simulink model "gg_plus_lc_platoon"  (R2019a)
settings: Solver=ode23t  StartTime=0.0  StopTime=70  FixedStep=0.1  MaxStep=0.01  RelTol=1e-3
InitFcn:
  | load vehStatesBus
libraries: simulink x120, powerlib_meascontrol x14, dspsigops x7, autolibshared x7
(part 7 of 7)

== system gg_plus_lc_platoon/p3/Virtual Vehicle Following/Virtual Leader Following ==
  eh : Inport
  ev : Inport  Port=2
  realInput : Inport  Port=3
  intReset : Inport  Port=4
  Anti-windup gain : Gain  Gain=sqrt(Ki/Kd)
  Gain : Gain  Gain=10
  Integrator : Integrator  ExternalReset=rising
  Integrator2 : Integrator  ExternalReset=rising
  Kd : Gain  Gain=Kd
  Ki : Gain  Gain=Ki
  Kp : Gain  Gain=Kp
  Saturation1 : Saturate  UpperLimit=maxHeadwayError  LowerLimit=minHeadwayError
  Scope : Scope  NumInputPorts=4
  Scope1 : Scope  NumInputPorts=2
  Sum : Sum  Inputs=|-+
  Sum1 : Sum  Inputs=+++
  Sum5 : Sum  Inputs=-+|
  Sum9 : Sum  Inputs=|+-
  u : Outport
  wires:
  Saturation1/1 -> Sum9/1, Scope1/1
  Sum9/1 -> Gain/1
  Gain/1 -> Integrator2/1
  ev/1 -> Kd/1
  Ki/1 -> Sum5/2
  Anti-windup gain/1 -> Sum5/1
  Sum5/1 -> Integrator/1
  Integrator/1 -> Sum1/1, Scope/1
  Kp/1 -> Scope/2, Sum1/2
  Kd/1 -> Scope/3, Sum1/3
  Integrator2/1 -> Kp/1, Ki/1, Scope1/2, Sum9/2
  eh/1 -> Saturation1/1
  Sum1/1 -> Sum/2, u/1, Scope/4
  realInput/1 -> Sum/1
  Sum/1 -> Anti-windup gain/1
  intReset/1 -> Integrator/2, Integrator2/2

== system gg_plus_lc_platoon/p3/findLeader/Subsystem ==
  ego : Inport
  all : Inport  Port=2
  Enable : EnablePort
  MATLAB Function : MATLAB Function  TreatAsAtomicUnit=on
  idx : Outport  InitialOutput=1
  wires:
  ego/1 -> MATLAB Function/1(ego)
  MATLAB Function/1(leaderIdx) -> idx/1
  all/1 -> MATLAB Function/2(allVehicles)

== system gg_plus_lc_platoon/p3/findLeader/farAwayVeh ==
  ego : Inport  OutDataTypeStr=Bus: vehStatesBus
  Bus Creator : BusCreator  Inputs=6  OutDataTypeStr=Bus: vehStatesBus  NonVirtualBus=on
  Bus Selector : BusSelector  OutputSignals=X,Y,Xdot,psi,u,delta
  Constant : Constant  Value=1000
  Sum : Sum  Inputs=++|
  Out1 : Outport  OutDataTypeStr=Bus: vehStatesBus
  wires:
  Bus Creator/1 -> Out1/1
  Constant/1 -> Sum/1
  Bus Selector/1 -> Sum/2  "<X>"
  ego/1 -> Bus Selector/1
  Sum/1 -> Bus Creator/1  "X"
  Bus Selector/2 -> Bus Creator/2  "<Y>"
  Bus Selector/3 -> Bus Creator/3  "<Xdot>"
  Bus Selector/4 -> Bus Creator/4  "<psi>"
  Bus Selector/5 -> Bus Creator/5  "<u>"
  Bus Selector/6 -> Bus Creator/6  "<delta>"

== system gg_plus_lc_platoon/p3/followerErrors/gapToFollower ==
  xf : Inport
  vf : Inport  Port=2
  xl : Inport  Port=3
  Multiply : Product
  Sum : Sum  Inputs=-+|
  Sum1 : Sum  Inputs=++|
  Sum2 : Sum  Inputs=+-|
  Sum3 : Sum  Inputs=|++
  d0 : Constant  Value=d0
  h : Constant  Value=h
  vLen : Constant  Value=lr+lf
  eh : Outport
  "gap " : Outport  Port=2
  wires:
  vLen/1 -> Sum1/1
  Multiply/1 -> Sum3/1
  Sum/1 -> "gap "/1, Sum2/1  "gap"
  xf/1 -> Sum1/2
  Sum3/1 -> Sum2/2  "desired  gap"
  vf/1 -> Multiply/1
  Sum1/1 -> Sum/1  "x (front bumber)"
  xl/1 -> Sum/2
  Sum2/1 -> eh/1
  h/1 -> Multiply/2  "time headway"
  d0/1 -> Sum3/2  "gap at  standstill"

== system gg_plus_lc_platoon/p3/safeErrors/Triggered Subsystem1 ==
  Trigger : TriggerPort  VariantControl=Variant
  Constant : Constant  Value=true  OutDataTypeStr=boolean
  Out1 : Outport  OutDataTypeStr=boolean  InitialOutput=0
  wires:
  Constant/1 -> Out1/1

== matlab function gg_plus_lc_platoon/Lo/Subsystem2/MATLAB Function ==
  data: strategy input; longAdjFlag output; posInPlatoon input; platoonState input
function longAdjFlag = startLongAdjustment(strategy, posInPlatoon, platoonState)

switch strategy
    case {1, 2}
        if posInPlatoon == 1
            longAdjFlag = true;
        else
            longAdjFlag = platoonState(posInPlatoon-1)>1;
        end
    case 3
        if posInPlatoon == length(platoonState)
            longAdjFlag = true;
        else
           longAdjFlag = platoonState(posInPlatoon+1)>4;
        end 
    otherwise
        error('Unknown strategy')
end

== matlab function gg_plus_lc_platoon/p1/Subsystem2/MATLAB Function ==
  data: strategy input; longAdjFlag output; posInPlatoon input; platoonState input
function longAdjFlag = startLongAdjustment(strategy, posInPlatoon, platoonState)

switch strategy
    case {1, 2}
        if posInPlatoon == 1
            longAdjFlag = true;
        else
            longAdjFlag = platoonState(posInPlatoon-1)>1;
        end
    case 3
        if posInPlatoon == length(platoonState)
            longAdjFlag = true;
        else
           longAdjFlag = platoonState(posInPlatoon+1)>4;
        end 
    otherwise
        error('Unknown strategy')
end

== stateflow chart gg_plus_lc_platoon/Lo/Virtual Vehicle Following/Chart ==
  state SpeedControlFreeFlow
    entry:
    state=2;
    during:
    u = uFreeFlowVelControl;
  state VehFollowing
    entry:
    state=0;
    during:
    u = uVehFoll;
  state SpeedControlMin
    entry:
    state = 1;
    during:
    u = uMinVelControl;
  (default) -> VehFollowing
  VehFollowing -> SpeedControlFreeFlow [order 2] : [~leaderWithinRange]
  SpeedControlFreeFlow -> VehFollowing : [leaderWithinRange]
  VehFollowing -> SpeedControlMin [order 1] : [(velDiff>=0) && (uVehFoll<0)]
  SpeedControlMin -> VehFollowing : [uVehFoll>=uMinVelControl]
  data: uFreeFlowVelControl input; leaderWithinRange input; uVehFoll input size=1; state output size=1; u output size=1; velDiff input size=1; uMinVelControl input double

== stateflow chart gg_plus_lc_platoon/Lo/controlChoice/ControlChoice ==
  state RegVehFoll
    during:
    data = regVehFollData;
  state AdjForLaneChange
    during:
    if ~xor(leaderInRange, vLeaderInRange)
    data = min(regVehFollData, longAdjustmentData);
    elseif vLeaderInRange
    data = longAdjustmentData;
    else
    data = regVehFollData;
    end
  (default) -> RegVehFoll
  RegVehFoll -> AdjForLaneChange : [state==1]
  data: state input; leaderInRange input; regVehFollData input; data output; longAdjustmentData input; vLeaderInRange input

== matlab function gg_plus_lc_platoon/Lo/findLeader/Subsystem/MATLAB Function ==
  data: ego input Bus: vehStatesBus; allVehicles input; leaderIdx output
function leaderIdx  = findLeader(ego, allVehicles)

nv = length(allVehicles);

leaderIdx = nv+1;

farAwayVehicle.X = ego.X + 10^4;
farAwayVehicle.Y = ego.Y;
farAwayVehicle.Xdot = ego.Xdot;
farAwayVehicle.u = 0;

leader = farAwayVehicle;
% For non lane changing vehicles, the leader is whoever is longitudinally
% closer and with any part of the body in the same lane.
% 1.8m (half lane) + 0.9m (half veh width)
for n = 1:nv
    if allVehicles(n).X>ego.X
        if abs(allVehicles(n).Y - ego.Y)<=2.7 && allVehicles(n).X<leader.X
            leaderIdx = n;
        end
    end
end

== matlab function gg_plus_lc_platoon/Lo/virtualVehiclesManager/MATLAB Function ==
  data: nVehicles input; longAdj input; lcFlag input; lcDone input; virtualLeaderIdx output; posInPlatoon input; lcStrategy input
function virtualLeaderIdx  = ...
    determineVirtualLeader(nVehicles, longAdj, lcFlag, lcDone, posInPlatoon, lcStrategy)

% Important assumption:
% The array of vehicles is ordered as [Ld, Fd, Lo, p1, ..., pN, Fo]

% To consider: would it be more organized to have two vehicle arrays (one 
% for each lane)?

if ~longAdj % vehicle not involved in LC
    virtualLeaderIdx = 1;
    return
end

if ~lcFlag% gap generating vehicle
    virtualLeaderIdx = nVehicles-1; % last platoon vehicle
    
else % lane changing vehicle
    switch lcStrategy
        case {1, 2} % synchronous, leader changes first
            if posInPlatoon == 1
                virtualLeaderIdx = 1;
            else
                virtualLeaderIdx = 3 + (posInPlatoon - 1);
            end
            
        case 3 % last veh changes first
            if ~lcDone
                virtualLeaderIdx = 1;
            else
                if posInPlatoon == 1
                    virtualLeaderIdx = 1;
                else
                    virtualLeaderIdx = 3 + (posInPlatoon - 1);
                end
            end
            
        otherwise
            error('[determineVirtualLeader in Simulink model] Unknown lane changing strategy]')
    end
end

end

== matlab function gg_plus_lc_platoon/Lo/virtualVehiclesManager/MATLAB Function1 ==
  data: nVehicles input; longAdj input; lcFlag input; posInPlatoon input; lcStrategy input; virtualFollowerIdx output
function virtualFollowerIdx  = ...
    determineVirtualFollower(nVehicles, longAdj, lcFlag, posInPlatoon, lcStrategy)

% Important assumption:
% The array of vehicles is ordered as [Ld, Fd, Lo, p1, ..., pN, Fo]

% To consider: would it be more organized to have two vehicle arrays (one 
% for each lane)?

if ~longAdj % vehicle not involved in LC
    virtualFollowerIdx = nVehicles;
    return
end

if ~lcFlag% gap generating vehicle
    virtualFollowerIdx = nVehicles;
    
else % lane changing vehicle
    switch lcStrategy
        case {1, 2} % synchronous, leader changes first
            virtualFollowerIdx = 2;
        case 3 % last veh changes first
            if posInPlatoon == nVehicles-4
                virtualFollowerIdx = 2;
            else
                virtualFollowerIdx = 3 + (posInPlatoon + 1);
            end
        otherwise
            error('[determineVirtualFollower in Simulink model] Unknown lane changing strategy]')
    end
end

end

== matlab function gg_plus_lc_platoon/Fo/Subsystem2/MATLAB Function ==
  data: strategy input; longAdjFlag output; posInPlatoon input; platoonState input
function longAdjFlag = startLongAdjustment(strategy, posInPlatoon, platoonState)

switch strategy
    case {1, 2}
        if posInPlatoon == 1
            longAdjFlag = true;
        else
            longAdjFlag = platoonState(posInPlatoon-1)>1;
        end
    case 3
        if posInPlatoon == length(platoonState)
            longAdjFlag = true;
        else
           longAdjFlag = platoonState(posInPlatoon+1)>4;
        end 
    otherwise
        error('Unknown strategy')
end

== stateflow chart gg_plus_lc_platoon/Fo/Virtual Vehicle Following/Chart ==
  state SpeedControlFreeFlow
    entry:
    state=2;
    during:
    u = uFreeFlowVelControl;
  state VehFollowing
    entry:
    state=0;
    during:
    u = uVehFoll;
  state SpeedControlMin
    entry:
    state = 1;
    during:
    u = uMinVelControl;
  (default) -> VehFollowing
  VehFollowing -> SpeedControlFreeFlow [order 2] : [~leaderWithinRange]
  SpeedControlFreeFlow -> VehFollowing : [leaderWithinRange]
  VehFollowing -> SpeedControlMin [order 1] : [(velDiff>=0) && (uVehFoll<0)]
  SpeedControlMin -> VehFollowing : [uVehFoll>=uMinVelControl]
  data: uFreeFlowVelControl input; leaderWithinRange input; uVehFoll input size=1; state output size=1; u output size=1; velDiff input size=1; uMinVelControl input double

== stateflow chart gg_plus_lc_platoon/Fo/controlChoice/ControlChoice ==
  state RegVehFoll
    during:
    data = regVehFollData;
  state AdjForLaneChange
    during:
    if ~xor(leaderInRange, vLeaderInRange)
    data = min(regVehFollData, longAdjustmentData);
    elseif vLeaderInRange
    data = longAdjustmentData;
    else
    data = regVehFollData;
    end
  (default) -> RegVehFoll
  RegVehFoll -> AdjForLaneChange : [state==1]
  data: state input; leaderInRange input; regVehFollData input; data output; longAdjustmentData input; vLeaderInRange input

== matlab function gg_plus_lc_platoon/Fo/findLeader/Subsystem/MATLAB Function ==
  data: ego input Bus: vehStatesBus; allVehicles input; leaderIdx output
function leaderIdx  = findLeader(ego, allVehicles)

nv = length(allVehicles);

leaderIdx = nv+1;

farAwayVehicle.X = ego.X + 10^4;
farAwayVehicle.Y = ego.Y;
farAwayVehicle.Xdot = ego.Xdot;
farAwayVehicle.u = 0;

leader = farAwayVehicle;
% For non lane changing vehicles, the leader is whoever is longitudinally
% closer and with any part of the body in the same lane.
% 1.8m (half lane) + 0.9m (half veh width)
for n = 1:nv
    if allVehicles(n).X>ego.X
        if abs(allVehicles(n).Y - ego.Y)<=2.7 && allVehicles(n).X<leader.X
            leaderIdx = n;
        end
    end
end

== matlab function gg_plus_lc_platoon/Fo/virtualVehiclesManager/MATLAB Function ==
  data: nVehicles input; longAdj input; lcFlag input; lcDone input; virtualLeaderIdx output; posInPlatoon input; lcStrategy input
function virtualLeaderIdx  = ...
    determineVirtualLeader(nVehicles, longAdj, lcFlag, lcDone, posInPlatoon, lcStrategy)

% Important assumption:
% The array of vehicles is ordered as [Ld, Fd, Lo, p1, ..., pN, Fo]

% To consider: would it be more organized to have two vehicle arrays (one 
% for each lane)?

if ~longAdj % vehicle not involved in LC
    virtualLeaderIdx = 1;
    return
end

if ~lcFlag% gap generating vehicle
    virtualLeaderIdx = nVehicles-1; % last platoon vehicle
    
else % lane changing vehicle
    switch lcStrategy
        case {1, 2} % synchronous, leader changes first
            if posInPlatoon == 1
                virtualLeaderIdx = 1;
            else
                virtualLeaderIdx = 3 + (posInPlatoon - 1);
            end
            
        case 3 % last veh changes first
            if ~lcDone
                virtualLeaderIdx = 1;
            else
                if posInPlatoon == 1
                    virtualLeaderIdx = 1;
                else
                    virtualLeaderIdx = 3 + (posInPlatoon - 1);
                end
            end
            
        otherwise
            error('[determineVirtualLeader in Simulink model] Unknown lane changing strategy]')
    end
end

end

== matlab function gg_plus_lc_platoon/Fo/virtualVehiclesManager/MATLAB Function1 ==
  data: nVehicles input; longAdj input; lcFlag input; posInPlatoon input; lcStrategy input; virtualFollowerIdx output
function virtualFollowerIdx  = ...
    determineVirtualFollower(nVehicles, longAdj, lcFlag, posInPlatoon, lcStrategy)

% Important assumption:
% The array of vehicles is ordered as [Ld, Fd, Lo, p1, ..., pN, Fo]

% To consider: would it be more organized to have two vehicle arrays (one 
% for each lane)?

if ~longAdj % vehicle not involved in LC
    virtualFollowerIdx = nVehicles;
    return
end

if ~lcFlag% gap generating vehicle
    virtualFollowerIdx = nVehicles;
    
else % lane changing vehicle
    switch lcStrategy
        case {1, 2} % synchronous, leader changes first
            virtualFollowerIdx = 2;
        case 3 % last veh changes first
            if posInPlatoon == nVehicles-4
                virtualFollowerIdx = 2;
            else
                virtualFollowerIdx = 3 + (posInPlatoon + 1);
            end
        otherwise
            error('[determineVirtualFollower in Simulink model] Unknown lane changing strategy]')
    end
end

end

== stateflow chart gg_plus_lc_platoon/p1/Virtual Vehicle Following/Chart ==
  state SpeedControlFreeFlow
    entry:
    state=2;
    during:
    u = uFreeFlowVelControl;
  state VehFollowing
    entry:
    state=0;
    during:
    u = uVehFoll;
  state SpeedControlMin
    entry:
    state = 1;
    during:
    u = uMinVelControl;
  (default) -> VehFollowing
  VehFollowing -> SpeedControlFreeFlow [order 2] : [~leaderWithinRange]
  SpeedControlFreeFlow -> VehFollowing : [leaderWithinRange]
  VehFollowing -> SpeedControlMin [order 1] : [(velDiff>=0) && (uVehFoll<0)]
  SpeedControlMin -> VehFollowing : [uVehFoll>=uMinVelControl]
  data: uFreeFlowVelControl input; leaderWithinRange input; uVehFoll input size=1; state output size=1; u output size=1; velDiff input size=1; uMinVelControl input double

== stateflow chart gg_plus_lc_platoon/p1/controlChoice/ControlChoice ==
  state RegVehFoll
    during:
    data = regVehFollData;
  state AdjForLaneChange
    during:
    if ~xor(leaderInRange, vLeaderInRange)
    data = min(regVehFollData, longAdjustmentData);
    elseif vLeaderInRange
    data = longAdjustmentData;
    else
    data = regVehFollData;
    end
  (default) -> RegVehFoll
  RegVehFoll -> AdjForLaneChange : [state==1]
  data: state input; leaderInRange input; regVehFollData input; data output; longAdjustmentData input; vLeaderInRange input

== matlab function gg_plus_lc_platoon/p1/findLeader/Subsystem/MATLAB Function ==
  data: ego input Bus: vehStatesBus; allVehicles input; leaderIdx output
function leaderIdx  = findLeader(ego, allVehicles)

nv = length(allVehicles);

leaderIdx = nv+1;

farAwayVehicle.X = ego.X + 10^4;
farAwayVehicle.Y = ego.Y;
farAwayVehicle.Xdot = ego.Xdot;
farAwayVehicle.u = 0;

leader = farAwayVehicle;
% For non lane changing vehicles, the leader is whoever is longitudinally
% closer and with any part of the body in the same lane.
% 1.8m (half lane) + 0.9m (half veh width)
for n = 1:nv
    if allVehicles(n).X>ego.X
        if abs(allVehicles(n).Y - ego.Y)<=2.7 && allVehicles(n).X<leader.X
            leaderIdx = n;
        end
    end
end

== matlab function gg_plus_lc_platoon/p1/virtualVehiclesManager/MATLAB Function ==
  data: nVehicles input; longAdj input; lcFlag input; lcDone input; virtualLeaderIdx output; posInPlatoon input; lcStrategy input
function virtualLeaderIdx  = ...
    determineVirtualLeader(nVehicles, longAdj, lcFlag, lcDone, posInPlatoon, lcStrategy)

% Important assumption:
% The array of vehicles is ordered as [Ld, Fd, Lo, p1, ..., pN, Fo]

% To consider: would it be more organized to have two vehicle arrays (one 
% for each lane)?

if ~longAdj % vehicle not involved in LC
    virtualLeaderIdx = 1;
    return
end

if ~lcFlag% gap generating vehicle
    virtualLeaderIdx = nVehicles-1; % last platoon vehicle
    
else % lane changing vehicle
    switch lcStrategy
        case {1, 2} % synchronous, leader changes first
            if posInPlatoon == 1
                virtualLeaderIdx = 1;
            else
                virtualLeaderIdx = 3 + (posInPlatoon - 1);
            end
            
        case 3 % last veh changes first
            if ~lcDone
                virtualLeaderIdx = 1;
            else
                if posInPlatoon == 1
                    virtualLeaderIdx = 1;
                else
                    virtualLeaderIdx = 3 + (posInPlatoon - 1);
                end
            end
            
        otherwise
            error('[determineVirtualLeader in Simulink model] Unknown lane changing strategy]')
    end
end

end

== matlab function gg_plus_lc_platoon/p1/virtualVehiclesManager/MATLAB Function1 ==
  data: nVehicles input; longAdj input; lcFlag input; posInPlatoon input; lcStrategy input; virtualFollowerIdx output
function virtualFollowerIdx  = ...
    determineVirtualFollower(nVehicles, longAdj, lcFlag, posInPlatoon, lcStrategy)

% Important assumption:
% The array of vehicles is ordered as [Ld, Fd, Lo, p1, ..., pN, Fo]

% To consider: would it be more organized to have two vehicle arrays (one 
% for each lane)?

if ~longAdj % vehicle not involved in LC
    virtualFollowerIdx = nVehicles;
    return
end

if ~lcFlag% gap generating vehicle
    virtualFollowerIdx = nVehicles;
    
else % lane changing vehicle
    switch lcStrategy
        case {1, 2} % synchronous, leader changes first
            virtualFollowerIdx = 2;
        case 3 % last veh changes first
            if posInPlatoon == nVehicles-4
                virtualFollowerIdx = 2;
            else
                virtualFollowerIdx = 3 + (posInPlatoon + 1);
            end
        otherwise
            error('[determineVirtualFollower in Simulink model] Unknown lane changing strategy]')
    end
end

end

== matlab function gg_plus_lc_platoon/p2/Subsystem2/MATLAB Function ==
  data: strategy input; longAdjFlag output; posInPlatoon input; platoonState input
function longAdjFlag = startLongAdjustment(strategy, posInPlatoon, platoonState)

switch strategy
    case {1, 2}
        if posInPlatoon == 1
            longAdjFlag = true;
        else
            longAdjFlag = platoonState(posInPlatoon-1)>1;
        end
    case 3
        if posInPlatoon == length(platoonState)
            longAdjFlag = true;
        else
           longAdjFlag = platoonState(posInPlatoon+1)>4;
        end 
    otherwise
        error('Unknown strategy')
end

== stateflow chart gg_plus_lc_platoon/p2/Virtual Vehicle Following/Chart ==
  state SpeedControlFreeFlow
    entry:
    state=2;
    during:
    u = uFreeFlowVelControl;
  state VehFollowing
    entry:
    state=0;
    during:
    u = uVehFoll;
  state SpeedControlMin
    entry:
    state = 1;
    during:
    u = uMinVelControl;
  (default) -> VehFollowing
  VehFollowing -> SpeedControlFreeFlow [order 2] : [~leaderWithinRange]
  SpeedControlFreeFlow -> VehFollowing : [leaderWithinRange]
  VehFollowing -> SpeedControlMin [order 1] : [(velDiff>=0) && (uVehFoll<0)]
  SpeedControlMin -> VehFollowing : [uVehFoll>=uMinVelControl]
  data: uFreeFlowVelControl input; leaderWithinRange input; uVehFoll input size=1; state output size=1; u output size=1; velDiff input size=1; uMinVelControl input double

== stateflow chart gg_plus_lc_platoon/p2/controlChoice/ControlChoice ==
  state RegVehFoll
    during:
    data = regVehFollData;
  state AdjForLaneChange
    during:
    if ~xor(leaderInRange, vLeaderInRange)
    data = min(regVehFollData, longAdjustmentData);
    elseif vLeaderInRange
    data = longAdjustmentData;
    else
    data = regVehFollData;
    end
  (default) -> RegVehFoll
  RegVehFoll -> AdjForLaneChange : [state==1]
  data: state input; leaderInRange input; regVehFollData input; data output; longAdjustmentData input; vLeaderInRange input

== matlab function gg_plus_lc_platoon/p2/findLeader/Subsystem/MATLAB Function ==
  data: ego input Bus: vehStatesBus; allVehicles input; leaderIdx output
function leaderIdx  = findLeader(ego, allVehicles)

nv = length(allVehicles);

leaderIdx = nv+1;

farAwayVehicle.X = ego.X + 10^4;
farAwayVehicle.Y = ego.Y;
farAwayVehicle.Xdot = ego.Xdot;
farAwayVehicle.u = 0;

leader = farAwayVehicle;
% For non lane changing vehicles, the leader is whoever is longitudinally
% closer and with any part of the body in the same lane.
% 1.8m (half lane) + 0.9m (half veh width)
for n = 1:nv
    if allVehicles(n).X>ego.X
        if abs(allVehicles(n).Y - ego.Y)<=2.7 && allVehicles(n).X<leader.X
            leaderIdx = n;
        end
    end
end

== matlab function gg_plus_lc_platoon/p2/virtualVehiclesManager/MATLAB Function ==
  data: nVehicles input; longAdj input; lcFlag input; lcDone input; virtualLeaderIdx output; posInPlatoon input; lcStrategy input
function virtualLeaderIdx  = ...
    determineVirtualLeader(nVehicles, longAdj, lcFlag, lcDone, posInPlatoon, lcStrategy)

% Important assumption:
% The array of vehicles is ordered as [Ld, Fd, Lo, p1, ..., pN, Fo]

% To consider: would it be more organized to have two vehicle arrays (one 
% for each lane)?

if ~longAdj % vehicle not involved in LC
    virtualLeaderIdx = 1;
    return
end

if ~lcFlag% gap generating vehicle
    virtualLeaderIdx = nVehicles-1; % last platoon vehicle
    
else % lane changing vehicle
    switch lcStrategy
        case {1, 2} % synchronous, leader changes first
            if posInPlatoon == 1
                virtualLeaderIdx = 1;
            else
                virtualLeaderIdx = 3 + (posInPlatoon - 1);
            end
            
        case 3 % last veh changes first
            if ~lcDone
                virtualLeaderIdx = 1;
            else
                if posInPlatoon == 1
                    virtualLeaderIdx = 1;
                else
                    virtualLeaderIdx = 3 + (posInPlatoon - 1);
                end
            end
            
        otherwise
            error('[determineVirtualLeader in Simulink model] Unknown lane changing strategy]')
    end
end

end

== matlab function gg_plus_lc_platoon/Fd/Subsystem2/MATLAB Function ==
  data: strategy input; longAdjFlag output; posInPlatoon input; platoonState input
function longAdjFlag = startLongAdjustment(strategy, posInPlatoon, platoonState)

switch strategy
    case {1, 2}
        if posInPlatoon == 1
            longAdjFlag = true;
        else
            longAdjFlag = platoonState(posInPlatoon-1)>1;
        end
    case 3
        if posInPlatoon == length(platoonState)
            longAdjFlag = true;
        else
           longAdjFlag = platoonState(posInPlatoon+1)>4;
        end 
    otherwise
        error('Unknown strategy')
end

== matlab function gg_plus_lc_platoon/p2/virtualVehiclesManager/MATLAB Function1 ==
  data: nVehicles input; longAdj input; lcFlag input; posInPlatoon input; lcStrategy input; virtualFollowerIdx output
function virtualFollowerIdx  = ...
    determineVirtualFollower(nVehicles, longAdj, lcFlag, posInPlatoon, lcStrategy)

% Important assumption:
% The array of vehicles is ordered as [Ld, Fd, Lo, p1, ..., pN, Fo]

% To consider: would it be more organized to have two vehicle arrays (one 
% for each lane)?

if ~longAdj % vehicle not involved in LC
    virtualFollowerIdx = nVehicles;
    return
end

if ~lcFlag% gap generating vehicle
    virtualFollowerIdx = nVehicles;
    
else % lane changing vehicle
    switch lcStrategy
        case {1, 2} % synchronous, leader changes first
            virtualFollowerIdx = 2;
        case 3 % last veh changes first
            if posInPlatoon == nVehicles-4
                virtualFollowerIdx = 2;
            else
                virtualFollowerIdx = 3 + (posInPlatoon + 1);
            end
        otherwise
            error('[determineVirtualFollower in Simulink model] Unknown lane changing strategy]')
    end
end

end

== matlab function gg_plus_lc_platoon/p3/Subsystem2/MATLAB Function ==
  data: strategy input; longAdjFlag output; posInPlatoon input; platoonState input
function longAdjFlag = startLongAdjustment(strategy, posInPlatoon, platoonState)

switch strategy
    case {1, 2}
        if posInPlatoon == 1
            longAdjFlag = true;
        else
            longAdjFlag = platoonState(posInPlatoon-1)>1;
        end
    case 3
        if posInPlatoon == length(platoonState)
            longAdjFlag = true;
        else
           longAdjFlag = platoonState(posInPlatoon+1)>4;
        end 
    otherwise
        error('Unknown strategy')
end

== stateflow chart gg_plus_lc_platoon/p3/Virtual Vehicle Following/Chart ==
  state SpeedControlFreeFlow
    entry:
    state=2;
    during:
    u = uFreeFlowVelControl;
  state VehFollowing
    entry:
    state=0;
    during:
    u = uVehFoll;
  state SpeedControlMin
    entry:
    state = 1;
    during:
    u = uMinVelControl;
  (default) -> VehFollowing
  VehFollowing -> SpeedControlFreeFlow [order 2] : [~leaderWithinRange]
  SpeedControlFreeFlow -> VehFollowing : [leaderWithinRange]
  VehFollowing -> SpeedControlMin [order 1] : [(velDiff>=0) && (uVehFoll<0)]
  SpeedControlMin -> VehFollowing : [uVehFoll>=uMinVelControl]
  data: uFreeFlowVelControl input; leaderWithinRange input; uVehFoll input size=1; state output size=1; u output size=1; velDiff input size=1; uMinVelControl input double

== stateflow chart gg_plus_lc_platoon/p3/controlChoice/ControlChoice ==
  state RegVehFoll
    during:
    data = regVehFollData;
  state AdjForLaneChange
    during:
    if ~xor(leaderInRange, vLeaderInRange)
    data = min(regVehFollData, longAdjustmentData);
    elseif vLeaderInRange
    data = longAdjustmentData;
    else
    data = regVehFollData;
    end
  (default) -> RegVehFoll
  RegVehFoll -> AdjForLaneChange : [state==1]
  data: state input; leaderInRange input; regVehFollData input; data output; longAdjustmentData input; vLeaderInRange input

== matlab function gg_plus_lc_platoon/p3/findLeader/Subsystem/MATLAB Function ==
  data: ego input Bus: vehStatesBus; allVehicles input; leaderIdx output
function leaderIdx  = findLeader(ego, allVehicles)

nv = length(allVehicles);

leaderIdx = nv+1;

farAwayVehicle.X = ego.X + 10^4;
farAwayVehicle.Y = ego.Y;
farAwayVehicle.Xdot = ego.Xdot;
farAwayVehicle.u = 0;

leader = farAwayVehicle;
% For non lane changing vehicles, the leader is whoever is longitudinally
% closer and with any part of the body in the same lane.
% 1.8m (half lane) + 0.9m (half veh width)
for n = 1:nv
    if allVehicles(n).X>ego.X
        if abs(allVehicles(n).Y - ego.Y)<=2.7 && allVehicles(n).X<leader.X
            leaderIdx = n;
        end
    end
end

== matlab function gg_plus_lc_platoon/p3/virtualVehiclesManager/MATLAB Function ==
  data: nVehicles input; longAdj input; lcFlag input; lcDone input; virtualLeaderIdx output; posInPlatoon input; lcStrategy input
function virtualLeaderIdx  = ...
    determineVirtualLeader(nVehicles, longAdj, lcFlag, lcDone, posInPlatoon, lcStrategy)

% Important assumption:
% The array of vehicles is ordered as [Ld, Fd, Lo, p1, ..., pN, Fo]

% To consider: would it be more organized to have two vehicle arrays (one 
% for each lane)?

if ~longAdj % vehicle not involved in LC
    virtualLeaderIdx = 1;
    return
end

if ~lcFlag% gap generating vehicle
    virtualLeaderIdx = nVehicles-1; % last platoon vehicle
    
else % lane changing vehicle
    switch lcStrategy
        case {1, 2} % synchronous, leader changes first
            if posInPlatoon == 1
                virtualLeaderIdx = 1;
            else
                virtualLeaderIdx = 3 + (posInPlatoon - 1);
            end
            
        case 3 % last veh changes first
            if ~lcDone
                virtualLeaderIdx = 1;
            else
                if posInPlatoon == 1
                    virtualLeaderIdx = 1;
                else
                    virtualLeaderIdx = 3 + (posInPlatoon - 1);
                end
            end
            
        otherwise
            error('[determineVirtualLeader in Simulink model] Unknown lane changing strategy]')
    end
end

end

== matlab function gg_plus_lc_platoon/p3/virtualVehiclesManager/MATLAB Function1 ==
  data: nVehicles input; longAdj input; lcFlag input; posInPlatoon input; lcStrategy input; virtualFollowerIdx output
function virtualFollowerIdx  = ...
    determineVirtualFollower(nVehicles, longAdj, lcFlag, posInPlatoon, lcStrategy)

% Important assumption:
% The array of vehicles is ordered as [Ld, Fd, Lo, p1, ..., pN, Fo]

% To consider: would it be more organized to have two vehicle arrays (one 
% for each lane)?

if ~longAdj % vehicle not involved in LC
    virtualFollowerIdx = nVehicles;
    return
end

if ~lcFlag% gap generating vehicle
    virtualFollowerIdx = nVehicles;
    
else % lane changing vehicle
    switch lcStrategy
        case {1, 2} % synchronous, leader changes first
            virtualFollowerIdx = 2;
        case 3 % last veh changes first
            if posInPlatoon == nVehicles-4
                virtualFollowerIdx = 2;
            else
                virtualFollowerIdx = 3 + (posInPlatoon + 1);
            end
        otherwise
            error('[determineVirtualFollower in Simulink model] Unknown lane changing strategy]')
    end
end

end

== stateflow chart gg_plus_lc_platoon/Fd/Virtual Vehicle Following/Chart ==
  state SpeedControlFreeFlow
    entry:
    state=2;
    during:
    u = uFreeFlowVelControl;
  state VehFollowing
    entry:
    state=0;
    during:
    u = uVehFoll;
  state SpeedControlMin
    entry:
    state = 1;
    during:
    u = uMinVelControl;
  (default) -> VehFollowing
  VehFollowing -> SpeedControlFreeFlow [order 2] : [~leaderWithinRange]
  SpeedControlFreeFlow -> VehFollowing : [leaderWithinRange]
  VehFollowing -> SpeedControlMin [order 1] : [(velDiff>=0) && (uVehFoll<0)]
  SpeedControlMin -> VehFollowing : [uVehFoll>=uMinVelControl]
  data: uFreeFlowVelControl input; leaderWithinRange input; uVehFoll input size=1; state output size=1; u output size=1; velDiff input size=1; uMinVelControl input double

== stateflow chart gg_plus_lc_platoon/Fd/controlChoice/ControlChoice ==
  state RegVehFoll
    during:
    data = regVehFollData;
  state AdjForLaneChange
    during:
    if ~xor(leaderInRange, vLeaderInRange)
    data = min(regVehFollData, longAdjustmentData);
    elseif vLeaderInRange
    data = longAdjustmentData;
    else
    data = regVehFollData;
    end
  (default) -> RegVehFoll
  RegVehFoll -> AdjForLaneChange : [state==1]
  data: state input; leaderInRange input; regVehFollData input; data output; longAdjustmentData input; vLeaderInRange input

== matlab function gg_plus_lc_platoon/Fd/findLeader/Subsystem/MATLAB Function ==
  data: ego input Bus: vehStatesBus; allVehicles input; leaderIdx output
function leaderIdx  = findLeader(ego, allVehicles)

nv = length(allVehicles);

leaderIdx = nv+1;

farAwayVehicle.X = ego.X + 10^4;
farAwayVehicle.Y = ego.Y;
farAwayVehicle.Xdot = ego.Xdot;
farAwayVehicle.u = 0;

leader = farAwayVehicle;
% For non lane changing vehicles, the leader is whoever is longitudinally
% closer and with any part of the body in the same lane.
% 1.8m (half lane) + 0.9m (half veh width)
for n = 1:nv
    if allVehicles(n).X>ego.X
        if abs(allVehicles(n).Y - ego.Y)<=2.7 && allVehicles(n).X<leader.X
            leaderIdx = n;
        end
    end
end

== matlab function gg_plus_lc_platoon/Fd/virtualVehiclesManager/MATLAB Function ==
  data: nVehicles input; longAdj input; lcFlag input; lcDone input; virtualLeaderIdx output; posInPlatoon input; lcStrategy input
function virtualLeaderIdx  = ...
    determineVirtualLeader(nVehicles, longAdj, lcFlag, lcDone, posInPlatoon, lcStrategy)

% Important assumption:
% The array of vehicles is ordered as [Ld, Fd, Lo, p1, ..., pN, Fo]

% To consider: would it be more organized to have two vehicle arrays (one 
% for each lane)?

if ~longAdj % vehicle not involved in LC
    virtualLeaderIdx = 1;
    return
end

if ~lcFlag% gap generating vehicle
    virtualLeaderIdx = nVehicles-1; % last platoon vehicle
    
else % lane changing vehicle
    switch lcStrategy
        case {1, 2} % synchronous, leader changes first
            if posInPlatoon == 1
                virtualLeaderIdx = 1;
            else
                virtualLeaderIdx = 3 + (posInPlatoon - 1);
            end
            
        case 3 % last veh changes first
            if ~lcDone
                virtualLeaderIdx = 1;
            else
                if posInPlatoon == 1
                    virtualLeaderIdx = 1;
                else
                    virtualLeaderIdx = 3 + (posInPlatoon - 1);
                end
            end
            
        otherwise
            error('[determineVirtualLeader in Simulink model] Unknown lane changing strategy]')
    end
end

end

== matlab function gg_plus_lc_platoon/Fd/virtualVehiclesManager/MATLAB Function1 ==
  data: nVehicles input; longAdj input; lcFlag input; posInPlatoon input; lcStrategy input; virtualFollowerIdx output
function virtualFollowerIdx  = ...
    determineVirtualFollower(nVehicles, longAdj, lcFlag, posInPlatoon, lcStrategy)

% Important assumption:
% The array of vehicles is ordered as [Ld, Fd, Lo, p1, ..., pN, Fo]

% To consider: would it be more organized to have two vehicle arrays (one 
% for each lane)?

if ~longAdj % vehicle not involved in LC
    virtualFollowerIdx = nVehicles;
    return
end

if ~lcFlag% gap generating vehicle
    virtualFollowerIdx = nVehicles;
    
else % lane changing vehicle
    switch lcStrategy
        case {1, 2} % synchronous, leader changes first
            virtualFollowerIdx = 2;
        case 3 % last veh changes first
            if posInPlatoon == nVehicles-4
                virtualFollowerIdx = 2;
            else
                virtualFollowerIdx = 3 + (posInPlatoon + 1);
            end
        otherwise
            error('[determineVirtualFollower in Simulink model] Unknown lane changing strategy]')
    end
end

end

== matlab function gg_plus_lc_platoon/Ld/Subsystem2/MATLAB Function ==
  data: strategy input; longAdjFlag output; posInPlatoon input; platoonState input
function longAdjFlag = startLongAdjustment(strategy, posInPlatoon, platoonState)

switch strategy
    case {1, 2}
        if posInPlatoon == 1
            longAdjFlag = true;
        else
            longAdjFlag = platoonState(posInPlatoon-1)>1;
        end
    case 3
        if posInPlatoon == length(platoonState)
            longAdjFlag = true;
        else
           longAdjFlag = platoonState(posInPlatoon+1)>4;
        end 
    otherwise
        error('Unknown strategy')
end

== stateflow chart gg_plus_lc_platoon/Ld/Virtual Vehicle Following/Chart ==
  state SpeedControlFreeFlow
    entry:
    state=2;
    during:
    u = uFreeFlowVelControl;
  state VehFollowing
    entry:
    state=0;
    during:
    u = uVehFoll;
  state SpeedControlMin
    entry:
    state = 1;
    during:
    u = uMinVelControl;
  (default) -> VehFollowing
  VehFollowing -> SpeedControlFreeFlow [order 2] : [~leaderWithinRange]
  SpeedControlFreeFlow -> VehFollowing : [leaderWithinRange]
  VehFollowing -> SpeedControlMin [order 1] : [(velDiff>=0) && (uVehFoll<0)]
  SpeedControlMin -> VehFollowing : [uVehFoll>=uMinVelControl]
  data: uFreeFlowVelControl input; leaderWithinRange input; uVehFoll input size=1; state output size=1; u output size=1; velDiff input size=1; uMinVelControl input double

== stateflow chart gg_plus_lc_platoon/Ld/controlChoice/ControlChoice ==
  state RegVehFoll
    during:
    data = regVehFollData;
  state AdjForLaneChange
    during:
    if ~xor(leaderInRange, vLeaderInRange)
    data = min(regVehFollData, longAdjustmentData);
    elseif vLeaderInRange
    data = longAdjustmentData;
    else
    data = regVehFollData;
    end
  (default) -> RegVehFoll
  RegVehFoll -> AdjForLaneChange : [state==1]
  data: state input; leaderInRange input; regVehFollData input; data output; longAdjustmentData input; vLeaderInRange input

== matlab function gg_plus_lc_platoon/Ld/findLeader/Subsystem/MATLAB Function ==
  data: ego input Bus: vehStatesBus; allVehicles input; leaderIdx output
function leaderIdx  = findLeader(ego, allVehicles)

nv = length(allVehicles);

leaderIdx = nv+1;

farAwayVehicle.X = ego.X + 10^4;
farAwayVehicle.Y = ego.Y;
farAwayVehicle.Xdot = ego.Xdot;
farAwayVehicle.u = 0;

leader = farAwayVehicle;
% For non lane changing vehicles, the leader is whoever is longitudinally
% closer and with any part of the body in the same lane.
% 1.8m (half lane) + 0.9m (half veh width)
for n = 1:nv
    if allVehicles(n).X>ego.X
        if abs(allVehicles(n).Y - ego.Y)<=2.7 && allVehicles(n).X<leader.X
            leaderIdx = n;
        end
    end
end

== matlab function gg_plus_lc_platoon/Ld/virtualVehiclesManager/MATLAB Function ==
  data: nVehicles input; longAdj input; lcFlag input; lcDone input; virtualLeaderIdx output; posInPlatoon input; lcStrategy input
function virtualLeaderIdx  = ...
    determineVirtualLeader(nVehicles, longAdj, lcFlag, lcDone, posInPlatoon, lcStrategy)

% Important assumption:
% The array of vehicles is ordered as [Ld, Fd, Lo, p1, ..., pN, Fo]

% To consider: would it be more organized to have two vehicle arrays (one 
% for each lane)?

if ~longAdj % vehicle not involved in LC
    virtualLeaderIdx = 1;
    return
end

if ~lcFlag% gap generating vehicle
    virtualLeaderIdx = nVehicles-1; % last platoon vehicle
    
else % lane changing vehicle
    switch lcStrategy
        case {1, 2} % synchronous, leader changes first
            if posInPlatoon == 1
                virtualLeaderIdx = 1;
            else
                virtualLeaderIdx = 3 + (posInPlatoon - 1);
            end
            
        case 3 % last veh changes first
            if ~lcDone
                virtualLeaderIdx = 1;
            else
                if posInPlatoon == 1
                    virtualLeaderIdx = 1;
                else
                    virtualLeaderIdx = 3 + (posInPlatoon - 1);
                end
            end
            
        otherwise
            error('[determineVirtualLeader in Simulink model] Unknown lane changing strategy]')
    end
end

end

== matlab function gg_plus_lc_platoon/Ld/virtualVehiclesManager/MATLAB Function1 ==
  data: nVehicles input; longAdj input; lcFlag input; posInPlatoon input; lcStrategy input; virtualFollowerIdx output
function virtualFollowerIdx  = ...
    determineVirtualFollower(nVehicles, longAdj, lcFlag, posInPlatoon, lcStrategy)

% Important assumption:
% The array of vehicles is ordered as [Ld, Fd, Lo, p1, ..., pN, Fo]

% To consider: would it be more organized to have two vehicle arrays (one 
% for each lane)?

if ~longAdj % vehicle not involved in LC
    virtualFollowerIdx = nVehicles;
    return
end

if ~lcFlag% gap generating vehicle
    virtualFollowerIdx = nVehicles;
    
else % lane changing vehicle
    switch lcStrategy
        case {1, 2} % synchronous, leader changes first
            virtualFollowerIdx = 2;
        case 3 % last veh changes first
            if posInPlatoon == nVehicles-4
                virtualFollowerIdx = 2;
            else
                virtualFollowerIdx = 3 + (posInPlatoon + 1);
            end
        otherwise
            error('[determineVirtualFollower in Simulink model] Unknown lane changing strategy]')
    end
end

end
